simulink model "bille_synthese_CDRE"  (R2019b)
settings: Solver=ode45  StartTime=0.0  StopTime=30  RelTol=1e-3  EnableMultiTasking=on
undefined symbols (not defined in the file): Ad, Bd, C, f, Fe, J, k, k1, k2, k3, kb, ki, kp, kpi, kv, Ld, lm, nm, rm, Te, tii
settings Model: ExtModeTrigMode=oneshot  ExtModeArmWhenConnect=off  Creator=khennouh  LastModifiedBy=lukas
settings DataIOCC: SaveFormat=Array  SignalLoggingSaveFormat=ModelDataLogs  ReturnWorkspaceOutputs=off
settings OptimizationCC: BlockReduction=off  BooleanDataType=off
settings DebuggingCC: SaveWithParameterizedLinksMsg=none  UnderspecifiedInitializationDetection=Classic  MergeDetectMultiDrivingBlocksExec=none  SignalResolutionControl=TryResolveAllWithWarning  MultiTaskDSMMsg=warning  MultiTaskCondExecSysMsg=none  ArithmeticOperatorsInVariantConditions=warning
settings HardwareCC: TargetUnknown=on
settings ModelReferenceCC: PropagateSignalLabelsOutOfModel=off
settings SFSimCC: SimUseLocalCustomCode=off  CustomCodeUndefinedFunction=UseInterfaceOnly
settings RTWCC: RTWUseLocalCustomCode=off
settings CodeAppCC: StateflowObjectComments=on
settings GRTTargetCC: TargetLangStandard=C89/C90 (ANSI)  CombineOutputUpdateFcns=off  GRTInterface=on

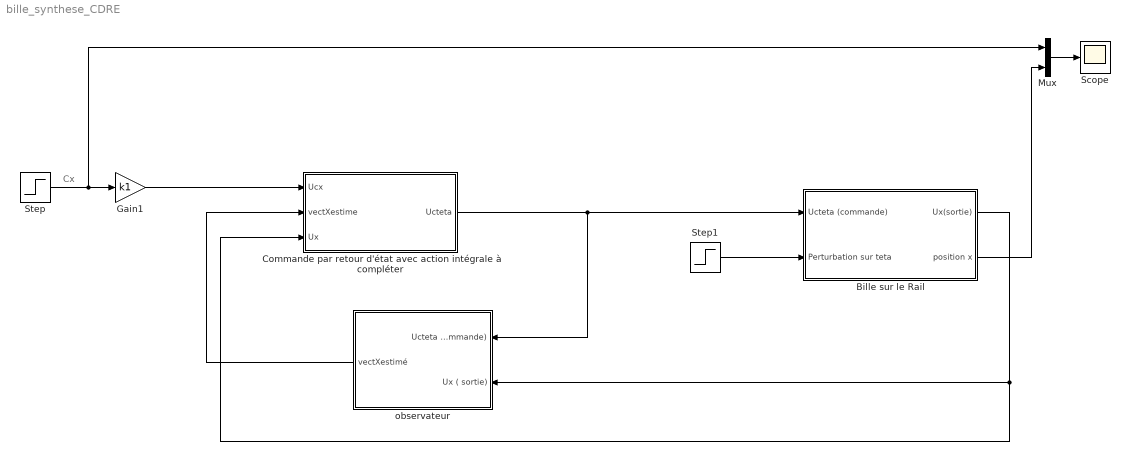
== system bille_synthese_CDRE ==
  note: Cx
  Bille sur le Rail : Subsystem
  Commande par retour d'état avec action intégrale à compléter : Subsystem
  Gain1 : Gain  Gain=k1
  Mux : Mux  Inputs=2
  Scope : Scope
  Step : Step  After=0.1  SampleTime=0
  Step1 : Step  Time=10  After=1*pi/180  SampleTime=0
  observateur : Subsystem
  wires:
  Step/1 -> Mux/1, Gain1/1
  Mux/1 -> Scope/1
  Commande par retour d'état avec action intégrale à compléter/1(Ucteta) -> Bille sur le Rail/1(Ucteta (commande)), observateur/1(Ucteta (commande))
  Gain1/1 -> Commande par retour d'état avec action intégrale à compléter/1(Ucx)
  observateur/1(vectXestimé) -> Commande par retour d'état avec action intégrale à compléter/2(vectXestime)
  Bille sur le Rail/1(Ux(sortie)) -> Commande par retour d'état avec action intégrale à compléter/3(Ux), observateur/2(Ux ( sortie))
  Step1/1 -> Bille sur le Rail/2(Perturbation sur teta)
  Bille sur le Rail/2(position x) -> Mux/2

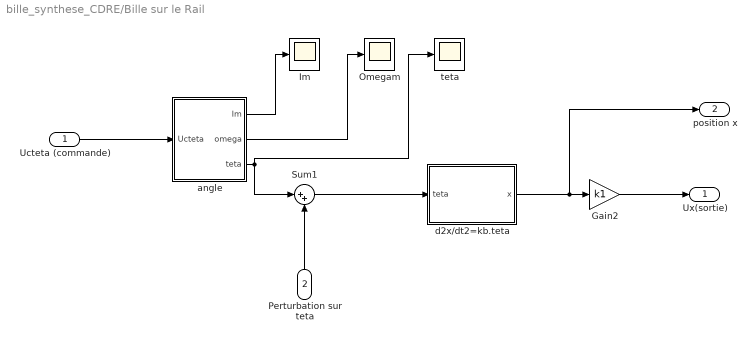
== system bille_synthese_CDRE/Bille sur le Rail ==
  Ucteta (commande) : Inport
  Perturbation sur teta : Inport  Port=2
  Gain2 : Gain  Gain=k1
  Im : Scope
  Omegam : Scope
  Sum1 : Sum  Inputs=|++  SaturateOnIntegerOverflow=on  InputSameDT=on  OutDataTypeStr=Inherit: Same as first input
  angle : Subsystem
  "d2x/dt2=kb.teta " : Subsystem
  teta : Scope
  Ux(sortie) : Outport  VectorParamsAs1DForOutWhenUnconnected=off
  position x : Outport  Port=2  VectorParamsAs1DForOutWhenUnconnected=off
  wires:
  angle/2(omega) -> Omegam/1
  Ucteta (commande)/1 -> angle/1(Ucteta)
  Perturbation sur teta/1 -> Sum1/2
  angle/3(teta) -> Sum1/1, teta/1
  angle/1(Im) -> Im/1
  Gain2/1 -> Ux(sortie)/1
  "d2x/dt2=kb.teta "/1(x) -> position x/1, Gain2/1
  Sum1/1 -> "d2x/dt2=kb.teta "/1(teta)

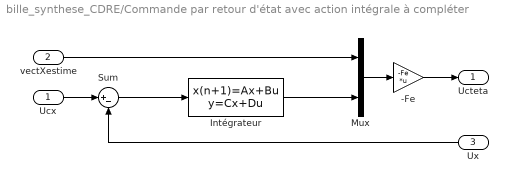
== system bille_synthese_CDRE/Commande par retour d'état avec action intégrale à compléter ==
  Ucx : Inport
  vectXestime : Inport  Port=2
  Ux : Inport  Port=3
  "-Fe " : Gain  Gain=-Fe  Multiplication=Matrix(K*u) (u vector)
  Intégrateur : DiscreteStateSpace  D=0  SampleTime=Te
  Mux : Mux  Inputs=2
  Sum : Sum  Inputs=|+-
  Ucteta : Outport  VectorParamsAs1DForOutWhenUnconnected=off
  wires:
  Intégrateur/1 -> Mux/2
  vectXestime/1 -> Mux/1
  Mux/1 -> "-Fe "/1
  Ucx/1 -> Sum/1
  Ux/1 -> Sum/2
  Sum/1 -> Intégrateur/1
  "-Fe "/1 -> Ucteta/1

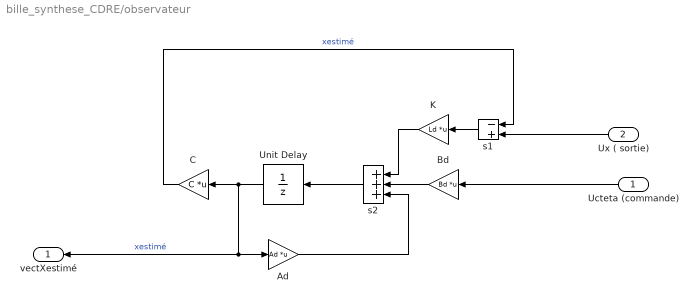
== system bille_synthese_CDRE/observateur ==
  Ucteta (commande) : Inport
  Ux ( sortie) : Inport  Port=2
  Ad : Gain  Gain=Ad  Multiplication=Matrix(K*u) (u vector)  SaturateOnIntegerOverflow=on  OutDataTypeStr=Inherit: Same as input  ParamDataTypeStr=Inherit: Same as input
  Bd : Gain  Gain=Bd  Multiplication=Matrix(K*u) (u vector)  SaturateOnIntegerOverflow=on  OutDataTypeStr=Inherit: Same as input  ParamDataTypeStr=Inherit: Same as input
  C : Gain  Gain=C  Multiplication=Matrix(K*u) (u vector)  SaturateOnIntegerOverflow=on  OutDataTypeStr=Inherit: Same as input  ParamDataTypeStr=Inherit: Same as input
  K : Gain  Gain=Ld  Multiplication=Matrix(K*u) (u vector)  SaturateOnIntegerOverflow=on  OutDataTypeStr=Inherit: Same as input  ParamDataTypeStr=Inherit: Same as input
  Unit Delay : UnitDelay  SampleTime=Te  HasFrameUpgradeWarning=on
  s1 : Sum  Inputs=-+  SaturateOnIntegerOverflow=on  InputSameDT=on  OutDataTypeStr=Inherit: Same as first input
  s2 : Sum  Inputs=+++  SaturateOnIntegerOverflow=on  InputSameDT=on  OutDataTypeStr=Inherit: Same as first input
  vectXestimé : Outport  VectorParamsAs1DForOutWhenUnconnected=off
  wires:
  Ux ( sortie)/1 -> s1/2
  Bd/1 -> s2/2
  s1/1 -> K/1
  C/1 -> s1/1  "xestimé"
  K/1 -> s2/1
  s2/1 -> Unit Delay/1
  Unit Delay/1 -> vectXestimé/1, Ad/1, C/1  "xestimé"
  Ad/1 -> s2/3
  Ucteta (commande)/1 -> Bd/1

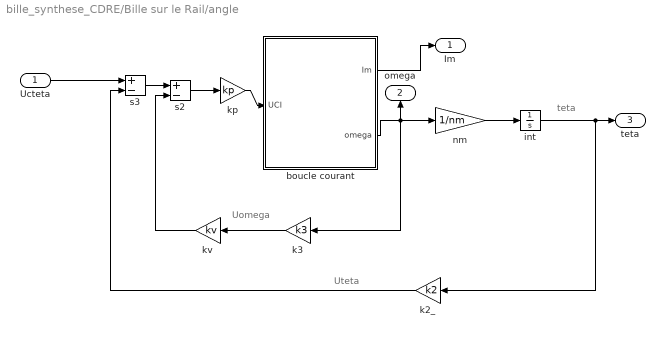
== system bille_synthese_CDRE/Bille sur le Rail/angle ==
  note: Uomega
  note: teta
  note: Uteta
  Ucteta : Inport
  boucle courant : Subsystem
  int : Integrator
  k2_ : Gain  Gain=k2  SaturateOnIntegerOverflow=on  OutDataTypeStr=Inherit: Same as input  ParamDataTypeStr=Inherit: Same as input
  k3 : Gain  Gain=k3  SaturateOnIntegerOverflow=on  OutDataTypeStr=Inherit: Same as input  ParamDataTypeStr=Inherit: Same as input
  kp : Gain  Gain=kp  SaturateOnIntegerOverflow=on  OutDataTypeStr=Inherit: Same as input  ParamDataTypeStr=Inherit: Same as input
  kv : Gain  Gain=kv  SaturateOnIntegerOverflow=on  OutDataTypeStr=Inherit: Same as input  ParamDataTypeStr=Inherit: Same as input
  nm : Gain  Gain=1/nm  SaturateOnIntegerOverflow=on  OutDataTypeStr=Inherit: Same as input  ParamDataTypeStr=Inherit: Same as input
  s2 : Sum  Inputs=+-  SaturateOnIntegerOverflow=on  InputSameDT=on  OutDataTypeStr=Inherit: Same as first input
  s3 : Sum  Inputs=+-  SaturateOnIntegerOverflow=on  InputSameDT=on  OutDataTypeStr=Inherit: Same as first input
  Im : Outport  VectorParamsAs1DForOutWhenUnconnected=off
  omega : Outport  Port=2  VectorParamsAs1DForOutWhenUnconnected=off
  teta : Outport  Port=3  VectorParamsAs1DForOutWhenUnconnected=off
  wires:
  kp/1 -> boucle courant/1(UCI)
  s2/1 -> kp/1
  s3/1 -> s2/1
  nm/1 -> int/1
  boucle courant/2(omega) -> nm/1, k3/1, omega/1
  k3/1 -> kv/1
  kv/1 -> s2/2
  int/1 -> k2_/1, teta/1
  k2_/1 -> s3/2
  boucle courant/1(Im) -> Im/1
  Ucteta/1 -> s3/1

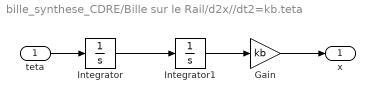
== system bille_synthese_CDRE/Bille sur le Rail/d2x//dt2=kb.teta  ==
  teta : Inport
  Gain : Gain  Gain=kb
  Integrator : Integrator
  Integrator1 : Integrator
  x : Outport  VectorParamsAs1DForOutWhenUnconnected=off
  wires:
  teta/1 -> Integrator/1
  Integrator/1 -> Integrator1/1
  Integrator1/1 -> Gain/1
  Gain/1 -> x/1

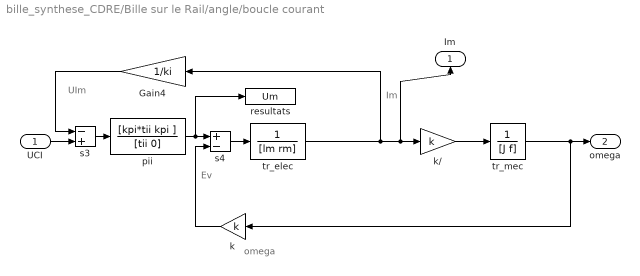
== system bille_synthese_CDRE/Bille sur le Rail/angle/boucle courant ==
  note: Im
  note: Ev
  note: UIm
  note: omega
  UCI : Inport
  Gain4 : Gain  Gain=1/ki  SaturateOnIntegerOverflow=on  OutDataTypeStr=Inherit: Same as input  ParamDataTypeStr=Inherit: Same as input
  k : Gain  Gain=k  SaturateOnIntegerOverflow=on  OutDataTypeStr=Inherit: Same as input  ParamDataTypeStr=Inherit: Same as input
  "k/ " : Gain  Gain=k  SaturateOnIntegerOverflow=on  OutDataTypeStr=Inherit: Same as input  ParamDataTypeStr=Inherit: Same as input
  pii : TransferFcn  Numerator=[kpi*tii kpi ]  Denominator=[tii 0]
  resultats : ToWorkspace  VariableName=Um
      settings: MaxDataPoints=20000
  s3 : Sum  Inputs=-+  SaturateOnIntegerOverflow=on  InputSameDT=on  OutDataTypeStr=Inherit: Same as first input
  s4 : Sum  Inputs=+-  SaturateOnIntegerOverflow=on  InputSameDT=on  OutDataTypeStr=Inherit: Same as first input
  tr_elec : TransferFcn  Denominator=[lm rm]
  tr_mec : TransferFcn  Denominator=[J f]
  Im : Outport  VectorParamsAs1DForOutWhenUnconnected=off
  omega : Outport  Port=2  VectorParamsAs1DForOutWhenUnconnected=off
  wires:
  s4/1 -> tr_elec/1
  Gain4/1 -> s3/1
  s3/1 -> pii/1
  k/1 -> s4/2
  "k/ "/1 -> tr_mec/1
  tr_mec/1 -> k/1, omega/1
  UCI/1 -> s3/2
  pii/1 -> s4/1, resultats/1
  tr_elec/1 -> Gain4/1, "k/ "/1, Im/1
